simulink subsystem "Day1_Scenario_1"  (R2024a)
settings: Solver=VariableStepAuto  StartTime=0.0  StopTime=10.0  RelTol=1e-3
libraries: CarMaker4SL x1
settings Model: Creator=junhyung.cha  LastModifiedBy=User

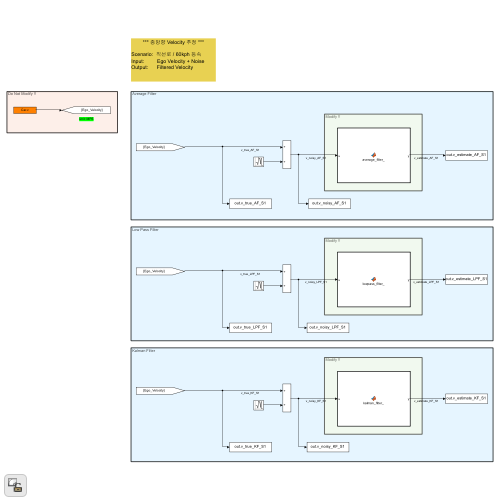
[thumbnail: Simulink's stored preview of the top-level diagram]
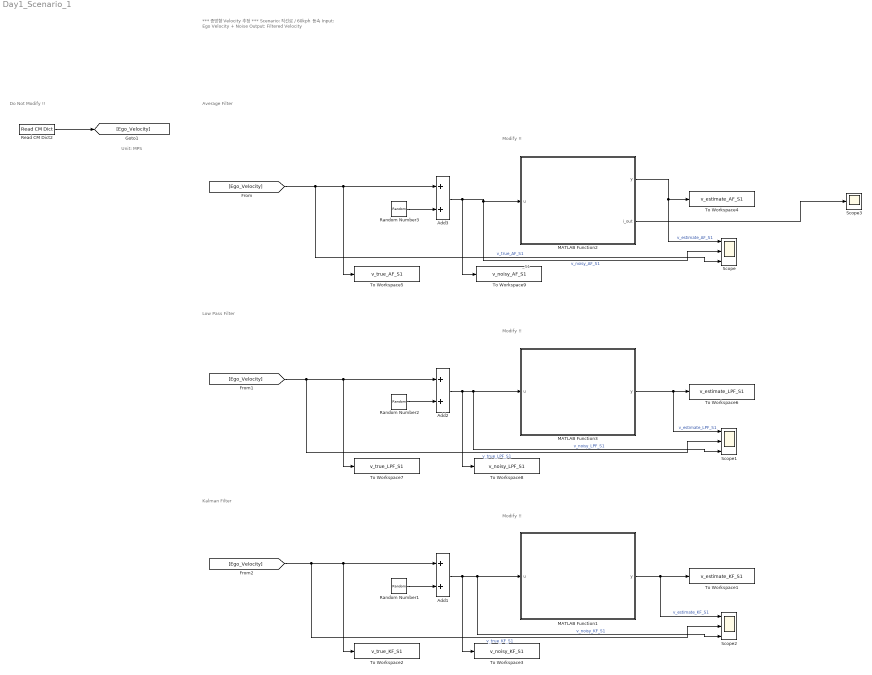
== system Day1_Scenario_1 ==
  note: _S1
  note: Modify !!
  note: Modify !!
  note: Modify !!
  note: Average Filter
  note: Low Pass Filter
  note: Kalman Filter
  note: *** 종방향 Velocity 추정 ***
      |
      | Scenario: 직선로 / 60kph 등속
      | Input: Ego Velocity + Noise
      | Output: Filtered Velocity
  note: Do Not Modify !!
  note: Unit: MPS
  Add1 : Sum
  Add2 : Sum
  Add3 : Sum
  MATLAB Function1 : MATLAB Function  TreatAsAtomicUnit=on
  MATLAB Function2 : MATLAB Function  TreatAsAtomicUnit=on
  MATLAB Function3 : MATLAB Function  TreatAsAtomicUnit=on
  Random Number1 : RandomNumber
  Random Number2 : RandomNumber
  Random Number3 : RandomNumber
  Read CM Dict2 : CarMaker4SL/Read CM Dict  xname=Car.v  xsync=off  xstime=Inherited
  Scope : Scope  NumInputPorts=3
  Scope1 : Scope  NumInputPorts=3
  Scope2 : Scope  NumInputPorts=3
  Scope3 : Scope
  To Workspace1 : ToWorkspace  VariableName=v_estimate_KF_S1  SaveFormat=Timeseries  SampleTime=-1
  To Workspace2 : ToWorkspace  VariableName=v_true_KF_S1  SaveFormat=Timeseries  SampleTime=-1
  To Workspace3 : ToWorkspace  VariableName=v_noisy_KF_S1  SaveFormat=Timeseries  SampleTime=-1
  To Workspace4 : ToWorkspace  VariableName=v_estimate_AF_S1  SaveFormat=Timeseries  SampleTime=-1
  To Workspace5 : ToWorkspace  VariableName=v_true_AF_S1  SaveFormat=Timeseries  SampleTime=-1
  To Workspace6 : ToWorkspace  VariableName=v_estimate_LPF_S1  SaveFormat=Timeseries  SampleTime=-1
  To Workspace7 : ToWorkspace  VariableName=v_true_LPF_S1  SaveFormat=Timeseries  SampleTime=-1
  To Workspace8 : ToWorkspace  VariableName=v_noisy_LPF_S1  SaveFormat=Timeseries  SampleTime=-1
  To Workspace9 : ToWorkspace  VariableName=v_noisy_AF_S1  SaveFormat=Timeseries  SampleTime=-1
  wires:
  Random Number2/1 -> Add2/2
  [Ego_Velocity] -> Add2/1, To Workspace7/1, Scope1/2  "v_true_LPF_S1"
  Add2/1 -> MATLAB Function3/1(u), Scope1/3, To Workspace8/1  "v_noisy_LPF_S1"
  MATLAB Function3/1(y) -> To Workspace6/1, Scope1/1  "v_estimate_LPF_S1"
  [Ego_Velocity] -> Add1/1, To Workspace2/1, Scope2/2  "v_true_KF_S1"
  MATLAB Function1/1(y) -> To Workspace1/1, Scope2/1  "v_estimate_KF_S1"
  Random Number1/1 -> Add1/2
  Add1/1 -> MATLAB Function1/1(u), Scope2/3, To Workspace3/1  "v_noisy_KF_S1"
  MATLAB Function2/1(y) -> To Workspace4/1, Scope/1  "v_estimate_AF_S1"
  Random Number3/1 -> Add3/2
  [Ego_Velocity] -> Add3/1, To Workspace5/1, Scope/3  "v_true_AF_S1"
  Add3/1 -> MATLAB Function2/1(u), Scope/2, To Workspace9/1  "v_noisy_AF_S1"
  Read CM Dict2/1 -> [Ego_Velocity]
  MATLAB Function2/2(i_out) -> Scope3/1

== matlab function Day1_Scenario_1/MATLAB Function2 ==
  settings: updateMethod=DISCRETE  sampleTime=0.05
  data: u input; y output; i_out output
function [y,i_out] = average_filter_(u)
    persistent i
    if isempty(i)
	    i = 0;
    end
    
    i = i+1;
    i_out = i;
    
    if i > 100
	    i=0;
    end
    y = 0;
end

== matlab function Day1_Scenario_1/MATLAB Function3 ==
  settings: updateMethod=DISCRETE  sampleTime=0.05
  data: u input; y output
function y = lowpass_filter_(u)
    y = 0;
    %#codegen
    % y[n] = alpha*u[n] + (1-alpha)*y[n-1]
    
    persistent alpha y_prev
    if isempty(alpha)
      alpha  = 0.2;    % Python 예제의 alpha
      y_prev = u;      % 초기 출력
    end
    
    % 지수 이동 평균
    y      = alpha*u + (1-alpha)*y_prev;
    y_prev = y;       % 상태 갱신
end

== matlab function Day1_Scenario_1/MATLAB Function1 ==
  settings: updateMethod=DISCRETE  sampleTime=0.05
  data: u input; y output
function y = kalman_filter_(u)
    y = 0;
%#codegen
% u : [측정값; 제어입력] 또는 스칼라(측정값만)
% y : 칼만 필터가 추정한 속도

  persistent A B C Q R P x_prev dt
  if isempty(A)
    % 1) Python 코드와 같은 파라미터로 초기화
    dt      = 0.1;    % step_time
    A       = 1.0;    % 상태 전이
    B       = dt;     % Python에서 B=step_time
    C       = 1.0;    % 관측 계수
    Q       = 0.01;   % 프로세스 잡음 분산
    R       = 1.0;    % 측정 잡음 분산
    P       = 10.0;   % 초기 오차 공분산
    x_prev  = u(1);   % 초기 상태 추정치: 첫 측정값
  end

  % 2) 입력 분리
  if numel(u) >= 2
    z       = u(1);  % 측정값
    input_u = u(2);  % 제어입력(가속도)
  else
    z       = u;     % 스칼라만 들어온 경우
    input_u = 0;     % 제어입력이 없으면 0
  end

  % — Prediction 단계 —
  x_pred = A * x_prev + B * input_u;
  P_pred = A * P * A + Q;

  % — Update 단계 —
  K      = P_pred * C / (C * P_pred * C + R);
  x_est  = x_pred + K * (z - C * x_pred);
  P      = (1 - K * C) * P_pred;

  % — 출력 및 내부 상태 저장 —
  y      = x_est;   % 블록 출력
  x_prev = x_est;   % 다음 스텝 예측을 위한 저장
end
